simulink model "Resistor_VoltageBased"  (R2018a)
settings: Solver=VariableStepAuto  StartTime=0.0  StopTime=10.0  RelTol=1e-3
libraries: Lib_PB_BuckConv_TMATS x1
settings Model: Creator=mebell  LastModifiedBy=mebell

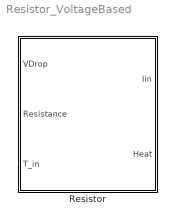
== system Resistor_VoltageBased ==
  Resistor : Subsystem  mask{TempIn=Celsius}
      mask prompts: TempIn "Input Units"
      mask init:
      | %Get current block name
      | block = gcb;
      | 
      | %Block under the mask(T_in inport and outport)
      | block2 = [block '/T_in'];
      | 
      | %Set T_in unit parameter to correct unit.
      | switch TempIn
      |     case 1 
      |         set_param(block2,'Unit','degF');
      |     case 2
      |         set_param(block2,'Unit','degC');
      |     case 3
      |         set_param(block2,'Unit','degR');
      |     case 4
      |         set_param(block2,'Unit','K');
      | end
      mask TypeOptions TempIn: Fahrenheit | Celsius | Rankine | Kelvin
      mask DialogControl Container4 Prompt: Parameters
      mask DialogControl Container6 Prompt: Temperature Units
      mask Display:
      | switch TempIn
      |     case 1
      |         port_label('input', 3, 'T_in (F)');
      |     case 2
      |         port_label('input', 3, 'T_in (C)');
      |     case 3
      |         port_label('input', 3, 'T_in (Ra)');
      |     case 4
      |         port_label('input', 3, 'T_in (K)');
      | end
      | 
      | port_label('input', 1, 'VDrop');
      | port_label('input', 2, 'Resistance');
      | 
      | 
      | port_label('output', 1, 'Iin');
      | port_label('output', 2, 'Heat');

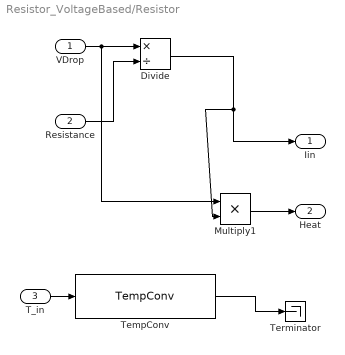
== system Resistor_VoltageBased/Resistor ==
  "VDrop " : Inport
  "Resistance " : Inport  Port=2
  T_in : Inport  Port=3  Unit=degC
  Divide : Product  Inputs=*/
  Multiply1 : Product
  "TempConv " : Lib_PB_BuckConv_TMATS/Buck Converter/TempConv 
  Terminator : Terminator
  Iin : Outport
  Heat : Outport  Port=2
  wires:
  Multiply1/1 -> Heat/1
  "VDrop "/1 -> Multiply1/1, Divide/1
  "Resistance "/1 -> Divide/2
  Divide/1 -> Multiply1/2, Iin/1
  T_in/1 -> "TempConv "/1
  "TempConv "/1 -> Terminator/1
